simulink model "sf_tlafter"  (Simulink 7.6)
settings: Solver=ode45  StartTime=0.0  StopTime=100  RelTol=1e-3
settings Model: Creator=The MathWorks Inc.  CovMetricSettings=dcmtr  ExtModeAutoUpdateStatusClock=off
settings OptimizationCC: BooleanDataType=off  InlineInvariantSignals=on  InitFltsAndDblsToZero=on  EfficientMapNaN2IntZero=off
settings DebuggingCC: SaveWithParameterizedLinksMsg=none  SignalResolutionControl=TryResolveAllWithWarning  SolverPrmCheckMsg=none  MultiTaskDSMMsg=warning  MultiTaskCondExecSysMsg=none  StrictBusMsg=None
settings HardwareCC: TargetUnknown=on
settings SFSimCC: SimParseCustomCode=off
settings RTWCC: IncludeERTFirstTime=on
settings GRTTargetCC: TargetFcnLib=ansi_tfl_tmw.mat

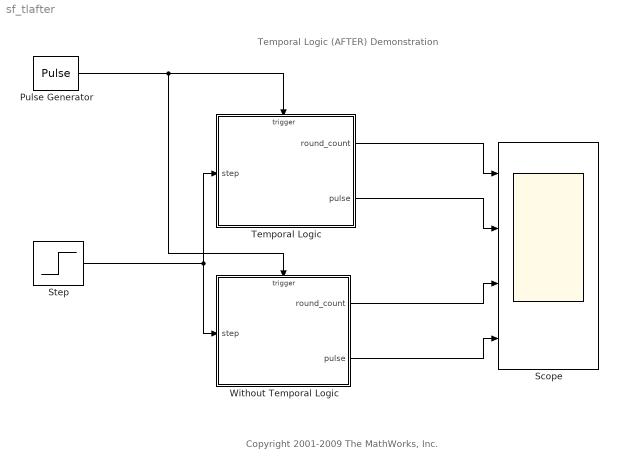
== system sf_tlafter ==
  note: Temporal Logic (AFTER) Demonstration
  note: Copyright 2001-2009 The MathWorks, Inc.
  Pulse Generator : DiscretePulseGenerator  PulseType=Time based  Period=1  PulseWidth=50
  Scope : Scope  NumInputPorts=4
      settings: TimeRange=100  YMin=0~-0.5~0~-0.5  YMax=6~1.5~6~1.5
  Step : Step  Time=60  SampleTime=0
  Temporal Logic : Stateflow chart  TreatAsAtomicUnit=on
  Without Temporal Logic : Stateflow chart  TreatAsAtomicUnit=on
  wires:
  Pulse Generator/1 -> Temporal Logic/Trigger, Without Temporal Logic/Trigger
  Temporal Logic/1(round_count) -> Scope/1
  Temporal Logic/2(pulse) -> Scope/2
  Without Temporal Logic/1(round_count) -> Scope/3
  Without Temporal Logic/2(pulse) -> Scope/4
  Step/1 -> Temporal Logic/1(step), Without Temporal Logic/1(step)

== stateflow chart Temporal Logic ==
  state Off
  state On
    en:pulse=1;
    exit:pulse=0;
  Off -> On : after(10,secs)[step<1]
  On -> Off : {round_count++;}
  (default) -> Off : {round_count=0;}
  data: round_count output double; pulse output double; step input double
  events: secs input RISING_EDGE_EVENT

== stateflow chart Without Temporal Logic ==
  state On [parallel]
    settings: executionOrder=1
    state A
      count_after=2;
      A -> A [order 1] : {count_after++;}
    state B
      entry: pulse=1;
      exit: pulse=0;
    A -> B [order 1] : [count_after>10 && step<1]
    B -> A : {round_count++;}
  (default) -> A
  data: round_count output double; count_after local double; pulse output double; step input double
  events: secs input RISING_EDGE_EVENT
